simulink model "TSCLAB_Modelv_1314"  (R2021a)
settings: Solver=VariableStepAuto  StartTime=0.0  StopTime=600  RelTol=1e-3
libraries: instrumentseriallib x3
settings Model: Creator=vasanza  LastModifiedBy=vasan
settings SolverCC: AlgebraicLoopSolver=TrustRegion
settings DebuggingCC: SFMachineParentedDataDiag=warning

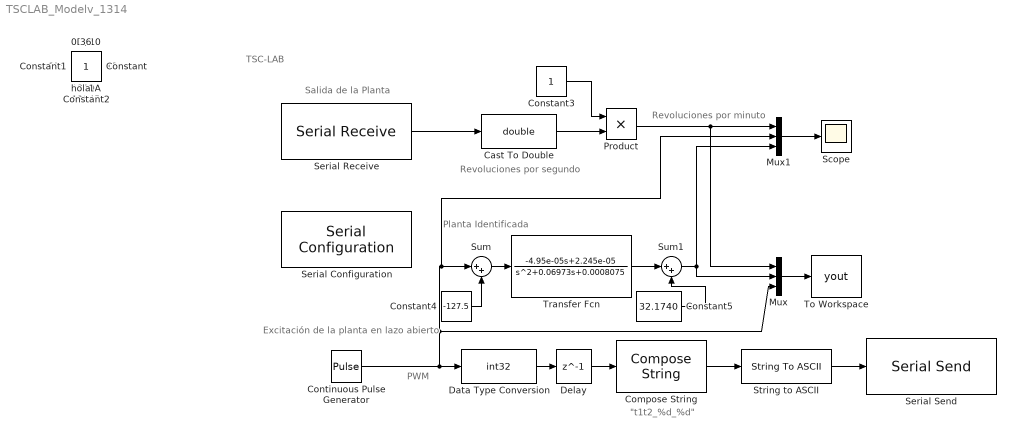
== system TSCLAB_Modelv_1314 ==
  note: "t1t2_%d_%d"
  note: PWM
  note: Excitación de la planta en lazo abierto
  note: Revoluciones por minuto
  note: Revoluciones por segundo
  note: Salida de la Planta
  note: TSC-LAB
  note: Planta Identificada
  Cast To Double : DataTypeConversion  OutDataTypeStr=double
  Compose String : ComposeString  Format="\"t1_%d\""
  Constant3 : Constant
  Constant4 : Constant  Value=-127.5
  Constant5 : Constant  Value=32.1740
  Continuous Pulse Generator : DiscretePulseGenerator  PulseType=Time based  Amplitude=255  Period=600  PulseWidth=50
  Data Type Conversion : DataTypeConversion  OutDataTypeStr=int32
  Delay : Delay  DelayLength=1  InitialCondition=0
  Mux : Mux  Inputs=3
  Mux1 : Mux  Inputs=3
  Product : Product
  Scope : Scope
  Serial Configuration : instrumentseriallib/Serial Configuration  Priority=-200000  Port=COM11  ComPort=COM11  BaudRate=115200  DataBits=8  Parity=none  StopBits=1  ByteOrder=little-endian  FlowControl=none  Timeout=10  SimulateUsing=Interpreted execution  BlockInModel=on
  Serial Receive : instrumentseriallib/Serial Receive  Port=COM11  ComPort=COM11  DataType=uint8  SaveDataType=uint8  ToggleHeader=off  Header=[]  ToggleTerminator=on  Terminator=<none>  CustomTerminator=[]  ToggleDataSize=on  DataSize=[1 1]  EnableBlockingMode=on  ActionDataUnavailable=Output last received value  ActionWhenDataUnavailable=Output last received value  CustomValue=0  SampleTime=0.999  SimulateUsing=Interpreted execution  BlockInModel=on
  Serial Send : instrumentseriallib/Serial Send  Port=COM11  ComPort=COM11  Header=[]  Terminator=<none>  CustomTerminator=[]  EnableBlockingMode=on  SimulateUsing=Interpreted execution  BlockInModel=on
  String to ASCII : StringToASCII
  Sum : Sum  Inputs=|++
  Sum1 : Sum  Inputs=|++
  To Workspace : ToWorkspace  VariableName=yout  SampleTime=-1
      settings: Save2DSignal=2-D array (concatenate along first dimension)
  Transfer Fcn : TransferFcn  Numerator=[-4.95e-05 2.245e-05]  Denominator=[1 0.06973 0.0008075]
  $ : Constant  IOType=siggen  Value=36
  , : Constant  IOType=siggen  Value=44
  {0,10,255,311,12345} (5 alike) : Constant  IOType=siggen
  0A : Constant  IOType=siggen  Value=10
  0D : Constant  IOType=siggen  Value=13
  13 : Constant  IOType=siggen  Value=13
  36 : Constant  IOType=siggen  Value=36
  Constant : Constant  IOType=siggen
  Constant1 : Constant  IOType=siggen
  Constant2 : Constant  IOType=siggen
  hola : Constant  IOType=siggen
  wires:
  Mux/1 -> To Workspace/1
  Data Type Conversion/1 -> Delay/1
  Serial Receive/1 -> Cast To Double/1
  Mux1/1 -> Scope/1
  Cast To Double/1 -> Product/2
  Constant3/1 -> Product/1
  Product/1 -> Mux/1, Mux1/1
  Delay/1 -> Compose String/1
  Compose String/1 -> String to ASCII/1
  String to ASCII/1 -> Serial Send/1
  Constant4/1 -> Sum/2
  Sum/1 -> Transfer Fcn/1
  Constant5/1 -> Sum1/2
  Continuous Pulse Generator/1 -> Data Type Conversion/1, Mux1/2, Sum/1, Mux/3
  Transfer Fcn/1 -> Sum1/1
  Sum1/1 -> Mux1/3, Mux/2
